simulink model "stable_model"  (R2021a)
settings: Solver=VariableStepAuto  StartTime=0.0  StopTime=10.0  RelTol=1e-3
values from neighbouring files (symbols this model uses):
  A = [0,0,1,0;0,0,0,1;0,(g*mp)/mc,-d1/mc,-d2/(L*mc);0,(g*(mc+mp))/(L*mc),-d1/(L*mc),-(d2*(mc+mp))/(L*L*mc*mp)]    [assgn_3.m]
  B = [0;0;1/mc;1/(L*mc)]    [assgn_3.m]
  K1 = lqr(A,B,Q,R)    [assgn_3.m]
  x0 = [0; 5*pi/180; 0 ; 0]    [assgn_3.m]
settings Model: Creator=hp  LastModifiedBy=hp

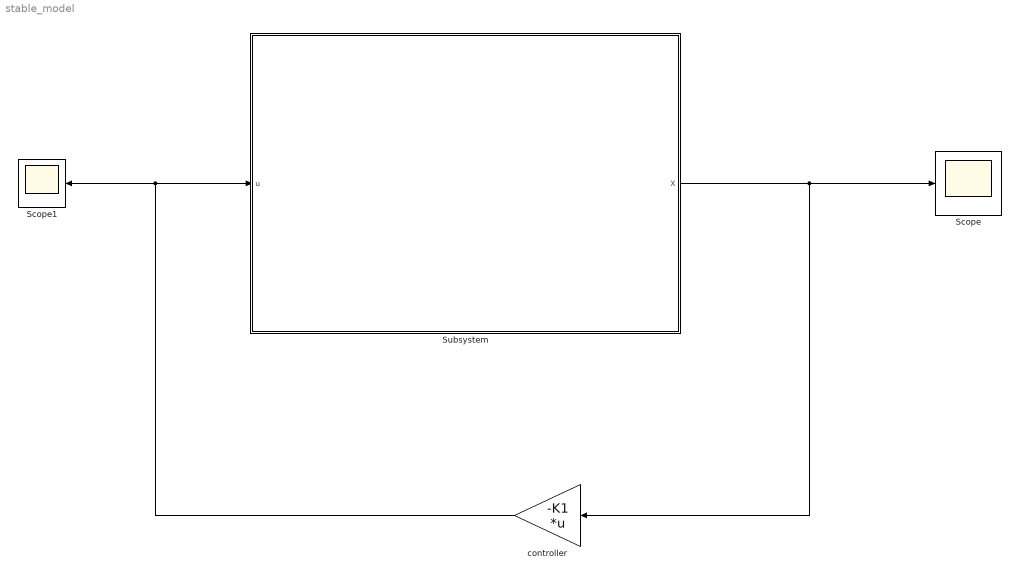
== system stable_model ==
  Scope : Scope
  Scope1 : Scope
  "Subsystem " : Subsystem
  controller : Gain  Gain=-K1  Multiplication=Matrix(K*u)
  wires:
  "Subsystem "/1(X) -> controller/1, Scope/1
  controller/1 -> "Subsystem "/1(u), Scope1/1

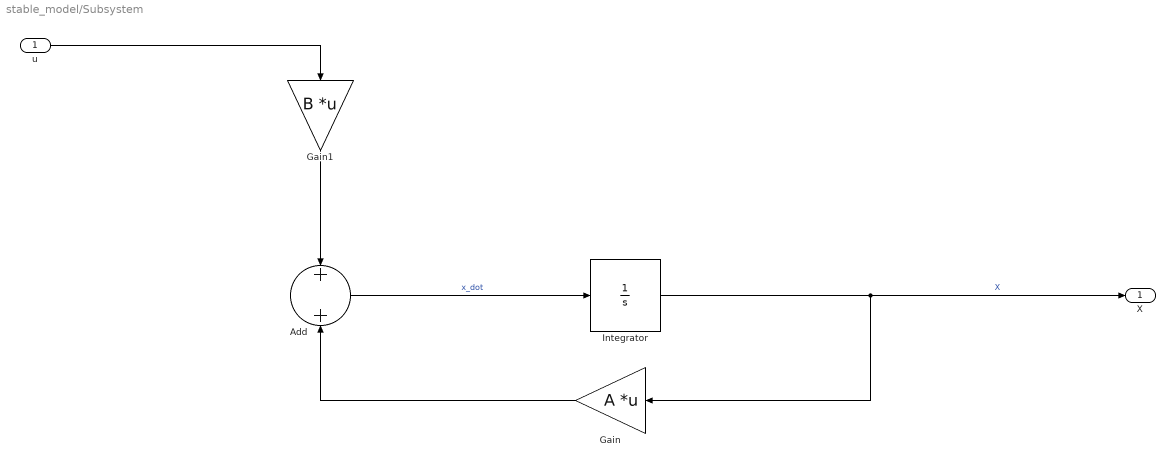
== system stable_model/Subsystem  ==
  u : Inport
  Add : Sum
  Gain : Gain  Gain=A  Multiplication=Matrix(K*u)
  Gain1 : Gain  Gain=B  Multiplication=Matrix(K*u)
  Integrator : Integrator  InitialCondition=x0
  X : Outport
  wires:
  u/1 -> Gain1/1
  Gain1/1 -> Add/1
  Add/1 -> Integrator/1  "x_dot"
  Gain/1 -> Add/2
  Integrator/1 -> X/1, Gain/1  "X"
